simulink model "positioning_system"  (R2020a)
settings: Solver=ode45  StartTime=0.0  StopTime=2  RelTol=1e-3
values from neighbouring files (symbols this model uses):
  C = 0.33e-06    (= 3.3e-07)    [main.m]
  d = 1    [main.m]
  E = 10    [main.m]
  Km = 5e-3    (= 0.005)    [main.m]
  Ks = 52.5    [main.m]
  P = 170e3    (= 170000)    [main.m]
  R = 10e3    (= 10000)    [main.m]
settings Model: Creator=ACER  LastModifiedBy=ACER

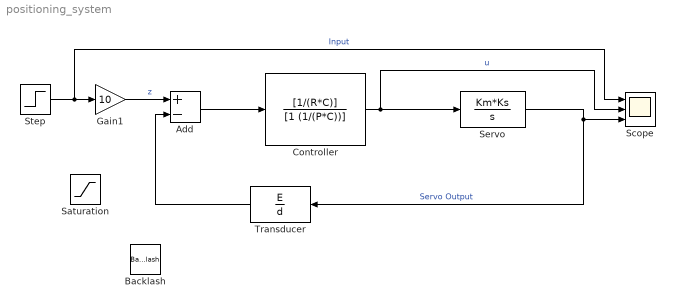
== system positioning_system ==
  Add : Sum  Inputs=+-
  Backlash : Backlash
  "Controller " : TransferFcn  Numerator=[1/(R*C)]  Denominator=[1 (1/(P*C))]
  Gain1 : Gain  Gain=10
  Saturation : Saturate
  Scope : Scope  NumInputPorts=3
  Servo : TransferFcn  Numerator=Km*Ks  Denominator=[1 0]
  Step : Step  After=0.5  SampleTime=0
  Transducer : TransferFcn  Numerator=E  Denominator=d
  wires:
  Step/1 -> Scope/1, Gain1/1  "Input"
  Gain1/1 -> Add/1  "z"
  Add/1 -> "Controller "/1
  "Controller "/1 -> Scope/2, Servo/1  "u"
  Transducer/1 -> Add/2
  Servo/1 -> Transducer/1, Scope/3  "Servo Output"
